simulink model "Admittance"  (R2020b)
settings: Solver=VariableStepAuto  StartTime=0.0  StopTime=5  RelTol=1e-3
values from neighbouring files (symbols this model uses):
  K = diag([2 2 2 0.1 0.1 0.1])    [parameters.m]
  KD = diag([ 500  500  135   0   0   400])    [parameters.m]
  KDt = 10*diag([18 18 18 18 18 18])    [parameters.m]
  KP = diag([ 1500 1700 2025  1   1   100])    [parameters.m]
  KPt = 100*diag([1 1 1 1 1 1])    [parameters.m]
  Md = diag([2 2 2 2 2 2])    [parameters.m]
  Mt = 0.75*diag([1 1 1 1 1 1])    [parameters.m]
libraries: robotcorelib x1, simulink x1, vrlib x1
settings Model: Creator=Edoardo  LastModifiedBy=Edoardo
settings SolverCC: AlgebraicLoopSolver=LineSearch

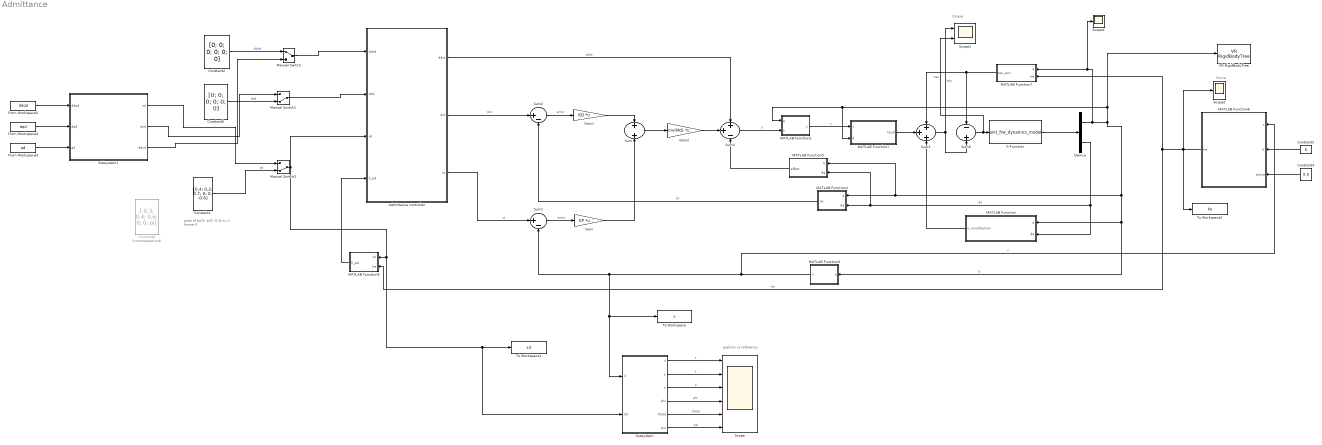
== system Admittance ==
  note: Force
  note: torque
  note: position vs reference
  note: pose of [pi/3 -pi/2 -0.1]
      | w.r.t. frame 0
  Admittance controller : Subsystem
  Constant1 : Constant  Value=[0.4; 0.2; 0.7; 0; 0; -0.6]  VectorParams1D=off
  Constant2 : Constant  Value=[0; 0; 0; 0; 0; 0]  VectorParams1D=off
  Constant3 : Constant  Value=K
  Constant4 : Constant  Value=0.5
  Constant5 : Constant  Value=[0; 0; 0; 0; 0; 0]  VectorParams1D=off
  Constant6 : Constant  Commented=on  Value=[-0.3; 0.4; 0.6; 0; 0; pi]  VectorParams1D=off
  Demux : Demux  Outputs=2
  From Workspace3 : FromWorkspace  VariableName=qd
  From Workspace4 : FromWorkspace  VariableName=dqd
  From Workspace5 : FromWorkspace  VariableName=ddqd
  Gain : Gain  Gain=KP  Multiplication=Matrix(K*u) (u vector)
  Gain1 : Gain  Gain=KD  Multiplication=Matrix(K*u) (u vector)
  Gain2 : Gain  Gain=inv(Md)  Multiplication=Matrix(K*u) (u vector)
  MATLAB Function : MATLAB Function  TreatAsAtomicUnit=on
  MATLAB Function1 : MATLAB Function  TreatAsAtomicUnit=on
  MATLAB Function2 : MATLAB Function  TreatAsAtomicUnit=on
  MATLAB Function3 : MATLAB Function  TreatAsAtomicUnit=on
  MATLAB Function4 : MATLAB Function  TreatAsAtomicUnit=on
  MATLAB Function5 : MATLAB Function  TreatAsAtomicUnit=on
  MATLAB Function6 : MATLAB Function  TreatAsAtomicUnit=on
  MATLAB Function7 : MATLAB Function  TreatAsAtomicUnit=on
  MATLAB Function9 : MATLAB Function  TreatAsAtomicUnit=on
  Manual Switch : ManualSwitch
  Manual Switch1 : ManualSwitch  CurrentSetting=0
  Manual Switch2 : ManualSwitch  CurrentSetting=0
  S-Function : S-Function  FunctionName=joint_frw_dynamics_model  Parameters=myRobot  SFunctionDeploymentMode=off  EnableBusSupport=off
  Scope : Scope  NumInputPorts=6
  Scope1 : Scope  NumInputPorts=2
  Scope2 : Scope
  Scope3 : Scope
  Subsystem : Subsystem
  Subsystem1 : Subsystem
  Sum : Sum
  Sum1 : Sum  Inputs=|+-
  Sum2 : Sum  Inputs=|+-
  Sum3 : Sum  Inputs=+++
  Sum4 : Sum  Inputs=++-
  Sum6 : Sum  Inputs=-+
  To Workspace : ToWorkspace  VariableName=x  SaveFormat=Timeseries  SampleTime=-1
  To Workspace1 : ToWorkspace  VariableName=xd  SaveFormat=Timeseries  SampleTime=-1
  To Workspace2 : ToWorkspace  VariableName=he  SaveFormat=Timeseries  SampleTime=-1
  VR RigidBodyTree : vrlib/VR RigidBodyTree  RBT=robot  useRBT=on  Ts=-1  ForceViewerOpen=on
      settings: SourceProductBaseCode=SL
  wires:
  Sum2/1 -> Gain1/1  "error"
  Sum1/1 -> Gain/1  "error"
  S-Function/1 -> Demux/1
  Sum3/1 -> Sum6/2, Scope1/1  "tau"
  Demux/2 -> MATLAB Function/2(dq), MATLAB Function4/2(dq), MATLAB Function5/2(dq)  "dq"
  Admittance controller/2(dxt) -> Sum2/1  "dxt"
  Demux/1 -> Scope3/1, MATLAB Function7/1(q), MATLAB Function4/1(q), MATLAB Function5/1(q), MATLAB Function3/1(q), MATLAB Function/1(q), VR RigidBodyTree/1, MATLAB Function2/1(q), MATLAB Function1/2(q)  "q"
  MATLAB Function2/1(y) -> MATLAB Function1/1(y)  "y"
  MATLAB Function4/1(dx) -> Sum2/2  "dx"
  Subsystem/1(x) -> Scope/1  "x"
  Subsystem/4(phi) -> Scope/4  "phi"
  Subsystem/6(psi) -> Scope/6  "psi"
  Subsystem/2(y) -> Scope/2  "y"
  Subsystem/5(theta) -> Scope/5  "theta"
  MATLAB Function3/1(x) -> MATLAB Function6/1(x), To Workspace/1, Subsystem/1(X), Sum1/2  "x"
  Admittance controller/3(xt) -> Sum1/1  "xt"
  Subsystem/3(z) -> Scope/3  "z"
  Constant4/1 -> MATLAB Function6/3(plane)
  Constant3/1 -> MATLAB Function6/2(K)
  MATLAB Function6/1(he) -> To Workspace2/1, MATLAB Function7/2(he), MATLAB Function9/2(he), Scope2/1  "he"
  MATLAB Function/1(n_contribution) -> Sum3/3
  MATLAB Function1/1(taud) -> Sum3/2
  MATLAB Function7/1(tau_env) -> Sum6/1, Sum3/1
  Sum4/1 -> MATLAB Function2/2(u)  "u"
  MATLAB Function5/1(effect) -> Sum4/3
  Gain1/1 -> Sum/1
  Gain/1 -> Sum/2
  Admittance controller/1(ddxt) -> Sum4/1  "ddxt"
  Gain2/1 -> Sum4/2
  Sum/1 -> Gain2/1
  Sum6/1 -> Scope1/2, S-Function/1  "tau"
  From Workspace5/1 -> Subsystem1/1(ddqd)
  Constant2/1 -> Manual Switch/1  "ddxd"
  From Workspace4/1 -> Subsystem1/2(dqd)
  Subsystem1/2(dxd) -> Manual Switch1/1
  Constant5/1 -> Manual Switch1/2  "dxd"
  From Workspace3/1 -> Subsystem1/3(qd)
  Constant1/1 -> Manual Switch2/2  "xd"
  Subsystem1/1(xd) -> Manual Switch2/1
  Manual Switch/1 -> Admittance controller/1(ddxd)
  Subsystem1/3(ddxd) -> Manual Switch/2
  Manual Switch2/1 -> To Workspace1/1, Subsystem/2(Xd), MATLAB Function9/1(xd), Admittance controller/3(xd)
  Manual Switch1/1 -> Admittance controller/2(dxd)
  MATLAB Function9/1(h_ed) -> Admittance controller/4(h_ed)

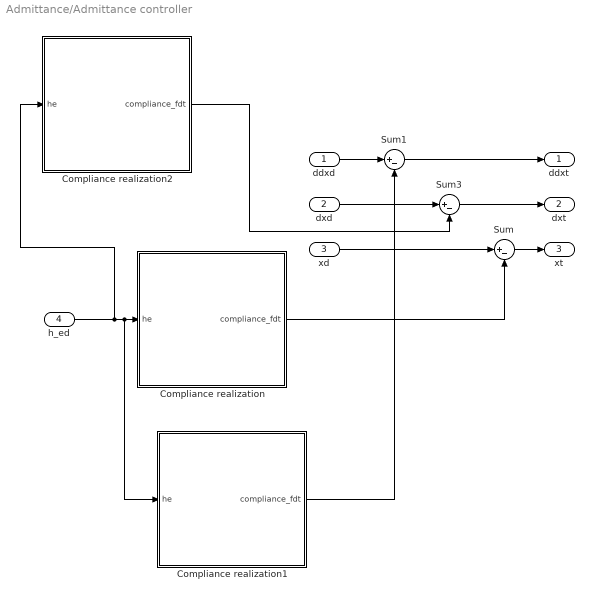
== system Admittance/Admittance controller ==
  ddxd : Inport
  dxd : Inport  Port=2
  xd : Inport  Port=3
  h_ed : Inport  Port=4
  Compliance realization : Subsystem
  Compliance realization1 : Subsystem
  Compliance realization2 : Subsystem
  Sum : Sum  Inputs=|+-
  Sum1 : Sum  Inputs=|+-
  Sum3 : Sum  Inputs=|+-
  ddxt : Outport
  dxt : Outport  Port=2
  xt : Outport  Port=3
  wires:
  xd/1 -> Sum/1
  dxd/1 -> Sum3/1
  ddxd/1 -> Sum1/1
  Sum3/1 -> dxt/1
  Sum/1 -> xt/1
  Sum1/1 -> ddxt/1
  Compliance realization/1(compliance_fdt) -> Sum/2
  h_ed/1 -> Compliance realization2/1(he), Compliance realization1/1(he), Compliance realization/1(he)
  Compliance realization2/1(compliance_fdt) -> Sum3/2
  Compliance realization1/1(compliance_fdt) -> Sum1/2

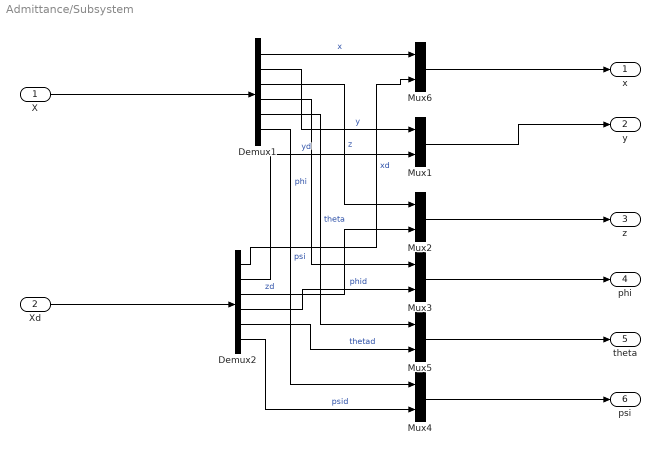
== system Admittance/Subsystem ==
  X : Inport
  Xd : Inport  Port=2
  Demux1 : Demux  Outputs=6
  Demux2 : Demux  Outputs=6
  Mux{1..6} (6 alike) : Mux  Inputs=2
  x : Outport
  y : Outport  Port=2
  z : Outport  Port=3
  phi : Outport  Port=4
  theta : Outport  Port=5
  psi : Outport  Port=6
  wires:
  Demux1/3 -> Mux2/1  "z"
  Demux1/4 -> Mux3/1  "phi"
  Demux2/3 -> Mux2/2  "zd"
  Mux2/1 -> z/1
  Demux2/1 -> Mux6/2  "xd"
  Demux1/5 -> Mux5/1  "theta"
  Mux1/1 -> y/1
  Demux1/6 -> Mux4/1  "psi"
  Demux1/1 -> Mux6/1  "x"
  Demux2/5 -> Mux5/2  "thetad"
  Demux2/6 -> Mux4/2  "psid"
  Demux1/2 -> Mux1/1  "y"
  Demux2/4 -> Mux3/2  "phid"
  Demux2/2 -> Mux1/2  "yd"
  Xd/1 -> Demux2/1
  X/1 -> Demux1/1
  Mux3/1 -> phi/1
  Mux5/1 -> theta/1
  Mux4/1 -> psi/1
  Mux6/1 -> x/1

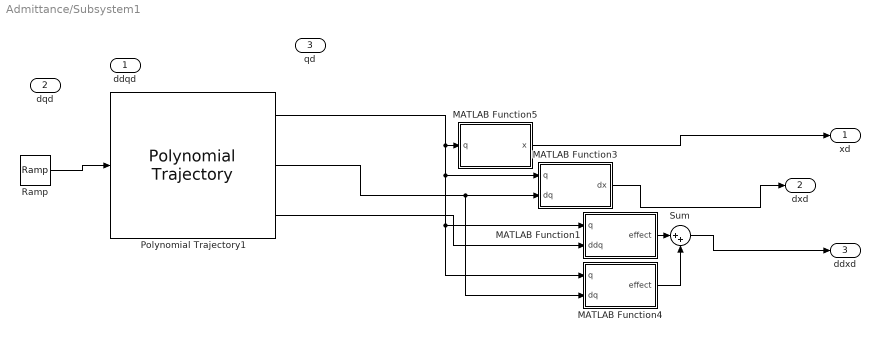
== system Admittance/Subsystem1 ==
  ddqd : Inport
  dqd : Inport  Port=2
  qd : Inport  Port=3
  MATLAB Function1 : MATLAB Function  TreatAsAtomicUnit=on
  MATLAB Function3 : MATLAB Function  TreatAsAtomicUnit=on
  MATLAB Function4 : MATLAB Function  TreatAsAtomicUnit=on
  MATLAB Function5 : MATLAB Function  TreatAsAtomicUnit=on
  Polynomial Trajectory1 : robotcorelib/Polynomial Trajectory  WaypointSource=Internal  Waypoints=[ pi/4, pi/4, pi/6;- pi/6,-pi/6, -pi/6; 0.1, 0.2, 0.1]  TimePoints=[ 0, 1.5, 5 ]  TimeInterval=[ 1, 4 ]  Method=Cubic Polynomial  ParameterSource=Internal  VelocityBoundaryCondition=zeros( 3, 3 )  AccelerationBoundaryCondition=zeros( 2, 5 )  SimulateUsing=Interpreted execution
      settings: SourceProductBaseCode=NV,RO,RR
  Ramp : simulink/Sources/Ramp  slope=1  start=0  InitialOutput=0
  Sum : Sum  Inputs=|++
  xd : Outport
  dxd : Outport  Port=2
  ddxd : Outport  Port=3
  wires:
  Polynomial Trajectory1/1 -> MATLAB Function4/1(q), MATLAB Function1/1(q), MATLAB Function3/1(q), MATLAB Function5/1(q)
  MATLAB Function4/1(effect) -> Sum/2
  Polynomial Trajectory1/2 -> MATLAB Function3/2(dq), MATLAB Function4/2(dq)
  MATLAB Function1/1(effect) -> Sum/1
  Polynomial Trajectory1/3 -> MATLAB Function1/2(ddq)
  MATLAB Function5/1(x) -> xd/1
  MATLAB Function3/1(dx) -> dxd/1
  Sum/1 -> ddxd/1
  Ramp/1 -> Polynomial Trajectory1/1

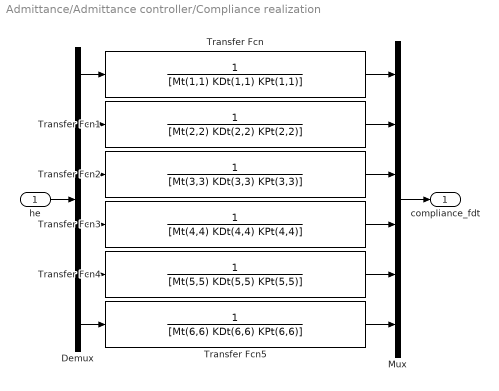
== system Admittance/Admittance controller/Compliance realization ==
  he : Inport
  Demux : Demux  Outputs=6
  Mux : Mux  Inputs=6
  Transfer Fcn : TransferFcn  Numerator=[0 0 1]  Denominator=[Mt(1,1) KDt(1,1) KPt(1,1)]
  Transfer Fcn1 : TransferFcn  Numerator=[0 0 1]  Denominator=[Mt(2,2) KDt(2,2) KPt(2,2)]
  Transfer Fcn2 : TransferFcn  Numerator=[0 0 1]  Denominator=[Mt(3,3) KDt(3,3) KPt(3,3)]
  Transfer Fcn3 : TransferFcn  Numerator=[0 0 1]  Denominator=[Mt(4,4) KDt(4,4) KPt(4,4)]
  Transfer Fcn4 : TransferFcn  Numerator=[0 0 1]  Denominator=[Mt(5,5) KDt(5,5) KPt(5,5)]
  Transfer Fcn5 : TransferFcn  Numerator=[0 0 1]  Denominator=[Mt(6,6) KDt(6,6) KPt(6,6)]
  compliance_fdt : Outport
  wires:
  Demux/5 -> Transfer Fcn4/1
  Transfer Fcn3/1 -> Mux/4
  Demux/4 -> Transfer Fcn3/1
  he/1 -> Demux/1
  Demux/1 -> Transfer Fcn/1
  Demux/6 -> Transfer Fcn5/1
  Transfer Fcn4/1 -> Mux/5
  Transfer Fcn2/1 -> Mux/3
  Mux/1 -> compliance_fdt/1
  Demux/2 -> Transfer Fcn1/1
  Transfer Fcn/1 -> Mux/1
  Demux/3 -> Transfer Fcn2/1
  Transfer Fcn5/1 -> Mux/6
  Transfer Fcn1/1 -> Mux/2

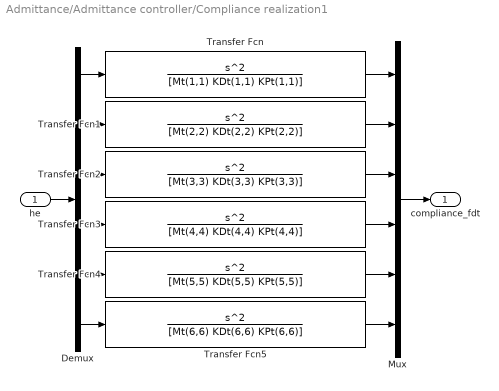
== system Admittance/Admittance controller/Compliance realization1 ==
  he : Inport
  Demux : Demux  Outputs=6
  Mux : Mux  Inputs=6
  Transfer Fcn : TransferFcn  Numerator=[1 0 0]  Denominator=[Mt(1,1) KDt(1,1) KPt(1,1)]
  Transfer Fcn1 : TransferFcn  Numerator=[1 0 0]  Denominator=[Mt(2,2) KDt(2,2) KPt(2,2)]
  Transfer Fcn2 : TransferFcn  Numerator=[1 0 0]  Denominator=[Mt(3,3) KDt(3,3) KPt(3,3)]
  Transfer Fcn3 : TransferFcn  Numerator=[1 0 0]  Denominator=[Mt(4,4) KDt(4,4) KPt(4,4)]
  Transfer Fcn4 : TransferFcn  Numerator=[1 0 0]  Denominator=[Mt(5,5) KDt(5,5) KPt(5,5)]
  Transfer Fcn5 : TransferFcn  Numerator=[1 0 0]  Denominator=[Mt(6,6) KDt(6,6) KPt(6,6)]
  compliance_fdt : Outport
  wires:
  Demux/5 -> Transfer Fcn4/1
  Transfer Fcn3/1 -> Mux/4
  Demux/4 -> Transfer Fcn3/1
  he/1 -> Demux/1
  Demux/1 -> Transfer Fcn/1
  Demux/6 -> Transfer Fcn5/1
  Transfer Fcn4/1 -> Mux/5
  Transfer Fcn2/1 -> Mux/3
  Mux/1 -> compliance_fdt/1
  Demux/2 -> Transfer Fcn1/1
  Transfer Fcn/1 -> Mux/1
  Demux/3 -> Transfer Fcn2/1
  Transfer Fcn5/1 -> Mux/6
  Transfer Fcn1/1 -> Mux/2

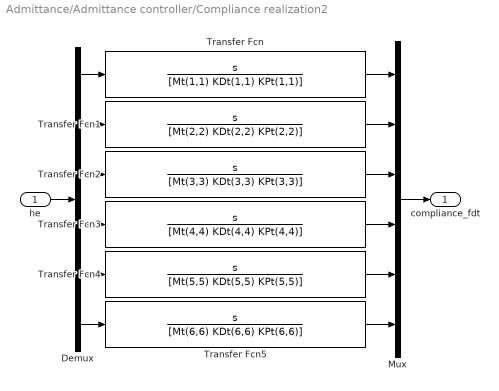
== system Admittance/Admittance controller/Compliance realization2 ==
  he : Inport
  Demux : Demux  Outputs=6
  Mux : Mux  Inputs=6
  Transfer Fcn : TransferFcn  Numerator=[0 1 0]  Denominator=[Mt(1,1) KDt(1,1) KPt(1,1)]
  Transfer Fcn1 : TransferFcn  Numerator=[0 1 0]  Denominator=[Mt(2,2) KDt(2,2) KPt(2,2)]
  Transfer Fcn2 : TransferFcn  Numerator=[0 1 0]  Denominator=[Mt(3,3) KDt(3,3) KPt(3,3)]
  Transfer Fcn3 : TransferFcn  Numerator=[0 1 0]  Denominator=[Mt(4,4) KDt(4,4) KPt(4,4)]
  Transfer Fcn4 : TransferFcn  Numerator=[0 1 0]  Denominator=[Mt(5,5) KDt(5,5) KPt(5,5)]
  Transfer Fcn5 : TransferFcn  Numerator=[0 1 0]  Denominator=[Mt(6,6) KDt(6,6) KPt(6,6)]
  compliance_fdt : Outport
  wires:
  Demux/5 -> Transfer Fcn4/1
  Transfer Fcn3/1 -> Mux/4
  Demux/4 -> Transfer Fcn3/1
  he/1 -> Demux/1
  Demux/1 -> Transfer Fcn/1
  Demux/6 -> Transfer Fcn5/1
  Transfer Fcn4/1 -> Mux/5
  Transfer Fcn2/1 -> Mux/3
  Mux/1 -> compliance_fdt/1
  Demux/2 -> Transfer Fcn1/1
  Transfer Fcn/1 -> Mux/1
  Demux/3 -> Transfer Fcn2/1
  Transfer Fcn5/1 -> Mux/6
  Transfer Fcn1/1 -> Mux/2

== matlab function Admittance/Subsystem1/MATLAB Function5 ==
  data: q input; x output
function x = K(q)

t1 = q(1);
t2 = q(2);
d3 = q(3);

K = [[ cos(t1 + t2), -sin(t1 + t2), 0, (3*cos(t1 + t2))/10 + (2*cos(t1))/5]
     [ sin(t1 + t2),  cos(t1 + t2), 0, (3*sin(t1 + t2))/10 + (2*sin(t1))/5]
     [            0,             0, 1,                            d3 + 2/5]
     [            0,             0, 0,                                   1]];

pos = K(1:3, 4);
ori = rotm2eul(K(1:3,1:3), 'ZYZ')';

x = [pos; ori];

== matlab function Admittance/MATLAB Function9 ==
  data: xd input; h_ed output; he input
function h_ed = TAT(xd,he)

orientation = xd(4:6);
h_ed = getTransformAnalytical(orientation)'*he;

== matlab function Admittance/MATLAB Function1 ==
  data: y input; taud output; q input size=3
function taud = B(y, q)

    taud = getBHatLagrangian(q)*y;

== matlab function Admittance/MATLAB Function ==
  data: q input size=3; n_contribution output; dq input size=3
function n_contribution = n(q,dq)
    n_contribution = getCHatLagrangian(q,dq)*dq + getGHatLagrangian(q);

== matlab function Admittance/MATLAB Function2 ==
  data: q input; u input; y output
function y = JA_inv(q,u)

y = pinv(getAnalyticalJacobian(q))*u;

== matlab function Admittance/MATLAB Function3 ==
  data: q input size=3; x output size=6
function x = K(q)

K = getDirectKinematics(q);

pos = K(1:3, 4);
rotm = K(1:3,1:3); 
ori = rotm2eul(rotm, 'ZYZ')';

x = [pos; ori];

== matlab function Admittance/MATLAB Function4 ==
  data: q input size=3; dx output size=6; dq input size=3
function dx = JA(q,dq)

dx = getAnalyticalJacobian(q)*dq;

== matlab function Admittance/MATLAB Function5 ==
  data: q input; effect output; dq input
function effect = dJA(q, dq)

    

effect = getDAnalyticalJacobian(q, dq)*dq;

== matlab function Admittance/MATLAB Function6 ==
  data: x input; he output; K input; plane input
function he = environment(x, K, plane)

% The robot is touching the environment! constrained motion
if x(3) >= plane
   
    xr = zeros(6,1);
    xr(3) = plane;
    
    % compute the forces 
    xe = zeros(6,1);
    xe(3) = x(3);

    he = K * (xe - xr);

% free motion
else
    
    he = zeros(6,1);
    
end

== matlab function Admittance/MATLAB Function7 ==
  data: q input; he input; tau_env output
function tau_env = JT(q, he)

tau_env = getJacobian(q)'*he;

== matlab function Admittance/Subsystem1/MATLAB Function3 ==
  data: q input; dx output; dq input
function dx = JA(q, dq)

dx = getAnalyticalJacobian(q)*dq;

== matlab function Admittance/Subsystem1/MATLAB Function1 ==
  data: q input; effect output; ddq input
function effect = JA(q, ddq)

effect = getAnalyticalJacobian(q)*ddq;

== matlab function Admittance/Subsystem1/MATLAB Function4 ==
  data: q input; effect output; dq input
function effect = dJA(q, dq)


effect = getDAnalyticalJacobian(q, dq)*dq;
